simulink model "CruiseCtrl_StateFeedback_Int"  (Simulink 8.3)
settings: Solver=ode45  StartTime=0.0  StopTime=40  MaxStep=0.01  RelTol=1e-3
values from neighbouring files (symbols this model uses):
  A = [[-1/tau 0];[1/m -rho*CD*Af*x2e/m]]    [CruiseCtrl_StateFeedback_Int_design.m]    (also in CruiseCtrl_StateFeedback_design.m; ej_01_CruiseCtrl_StateFeedback_design.m; ej_02_CruiseCtrl_StateFeedback_design.m)
  alpha = 2 * pi/180    (= 0.0349065850399)    [ej_01_CruiseCtrl_StateFeedback_design.m]    (also in ej_02_CruiseCtrl_StateFeedback_design.m)
  B1 = [B H]    [CruiseCtrl_StateFeedback_Int_design.m]    (also in CruiseCtrl_StateFeedback_design.m; ej_01_CruiseCtrl_StateFeedback_design.m; ej_02_CruiseCtrl_StateFeedback_design.m)
  C1 = eye(2)    [CruiseCtrl_StateFeedback_Int_design.m]    (also in CruiseCtrl_StateFeedback_design.m; ej_01_CruiseCtrl_StateFeedback_design.m; ej_02_CruiseCtrl_StateFeedback_design.m)
  D1 = zeros(2)    [CruiseCtrl_StateFeedback_Int_design.m]    (also in CruiseCtrl_StateFeedback_design.m; ej_01_CruiseCtrl_StateFeedback_design.m; ej_02_CruiseCtrl_StateFeedback_design.m)
  g = 9.82    [CruiseCtrl_StateFeedback_Int_design.m]    (also in CruiseCtrl_StateFeedback_design.m; ej_01_CruiseCtrl_StateFeedback_design.m; ej_02_CruiseCtrl_StateFeedback_design.m)
  Ku = v *  Wr_tilde * Wr^(-1)    [ej_02_CruiseCtrl_StateFeedback_design.m]
  ue = rw*x1e/k/r    (= 0.201)    [CruiseCtrl_StateFeedback_Int_design.m]    (also in CruiseCtrl_StateFeedback_design.m = 0.214125; ej_01_CruiseCtrl_StateFeedback_design.m = 0.214125; ej_02_CruiseCtrl_StateFeedback_design.m = 0.214125)
  x1e = 0.5*rho*CD*Af*x2e^2+m*g*f    (= 3216)    [CruiseCtrl_StateFeedback_Int_design.m]    (also in CruiseCtrl_StateFeedback_design.m = 3426; ej_01_CruiseCtrl_StateFeedback_design.m = 3426; ej_02_CruiseCtrl_StateFeedback_design.m = 3426)
  x2e = 15    [CruiseCtrl_StateFeedback_Int_design.m]    (also in CruiseCtrl_StateFeedback_design.m = 20; ej_01_CruiseCtrl_StateFeedback_design.m = 20; ej_02_CruiseCtrl_StateFeedback_design.m = 20)
settings Model: Creator=JonasMac  LastModifiedBy=rodralez  CovSFcnEnable=on
settings DataIOCC: SignalLoggingSaveFormat=Dataset
settings DebuggingCC: FrameProcessingCompatibilityMsg=error  StateNameClashWarn=none
settings GRTTargetCC: CombineOutputUpdateFcns=on  GRTInterface=off

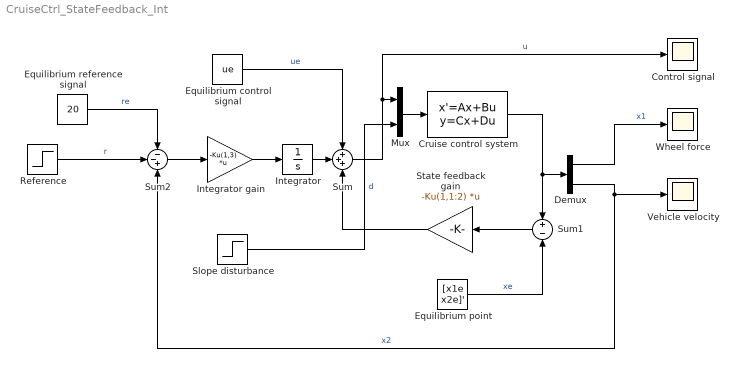
== system CruiseCtrl_StateFeedback_Int ==
  Control signal : Scope
      settings: TimeRange=auto  MaxDataPoints=5000  SaveName=control  YMin=-0.06478  YMax=2.15861  SampleTime=-1
  Cruise control system : StateSpace  A=A  B=B1  C=C1  D=D1
  Demux : Demux  Outputs=2
  Equilibrium control signal : Constant  Value=ue
  "Equilibrium point " : Constant  Value=[x1e x2e]'
  Equilibrium reference signal : Constant  Value=20
  Integrator : Integrator
  Integrator gain : Gain  Gain=-Ku(1,3)  Multiplication=Matrix(K*u)
  Mux : Mux  Inputs=2
  Reference : Step  After=5  SampleTime=0
  Slope disturbance : Step  Time=20  After=g*sin(alpha)  SampleTime=0
  State feedback gain : Gain  Gain=-Ku(1,1:2)  Multiplication=Matrix(K*u)
  Sum : Sum  Inputs=+++
  Sum1 : Sum  Inputs=+-
  Sum2 : Sum  Inputs=--+
  Vehicle velocity : Scope
      settings: TimeRange=auto  MaxDataPoints=5000  SaveName=velocity  YMin=19.35235  YMax=25.82882  SampleTime=-1
  Wheel force : Scope
      settings: TimeRange=auto  MaxDataPoints=5000  SaveToWorkspace=off  SaveName=ScopeData  YMin=-10  YMax=10  SampleTime=-1
  wires:
  Demux/1 -> Wheel force/1  "x1"
  Demux/2 -> Sum2/3, Vehicle velocity/1  "x2"
  Sum/1 -> Control signal/1, Mux/1  "u"
  Slope disturbance/1 -> Mux/2  "d"
  Integrator/1 -> Sum/2
  Equilibrium control signal/1 -> Sum/1  "ue"
  Cruise control system/1 -> Sum1/1, Demux/1
  Mux/1 -> Cruise control system/1
  State feedback gain/1 -> Sum/3
  Sum1/1 -> State feedback gain/1
  "Equilibrium point "/1 -> Sum1/2  "xe"
  Sum2/1 -> Integrator gain/1
  Integrator gain/1 -> Integrator/1
  Reference/1 -> Sum2/2  "r"
  Equilibrium reference signal/1 -> Sum2/1  "re"
